simulink model "simulink_chapter_1"  (R2020b)
settings: Solver=VariableStepAuto  StartTime=0.0  StopTime=10.0  RelTol=1e-3
undefined symbols (not defined in the file): c, k, m
libraries: simulink x1
settings Model: Creator=yosef  LastModifiedBy=yosef

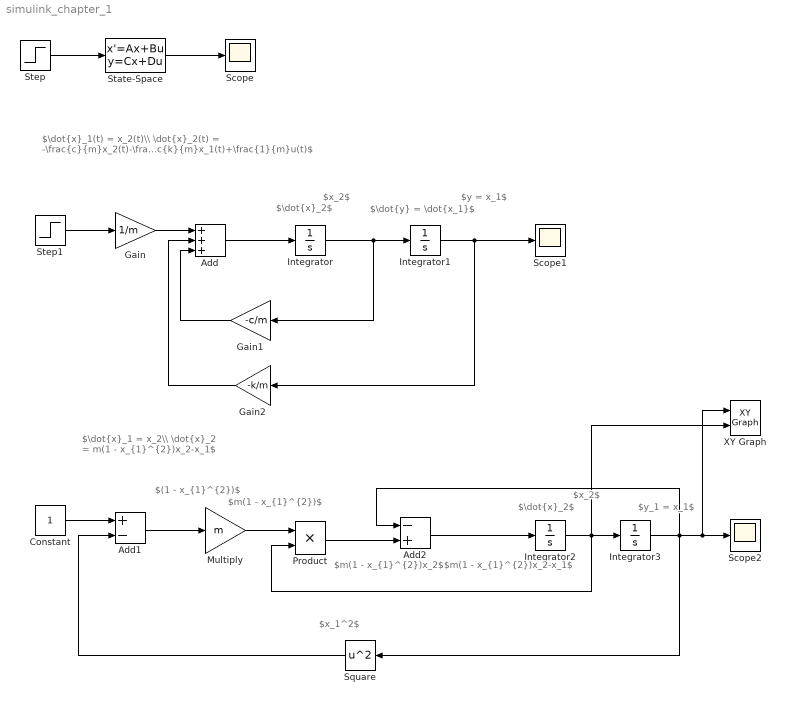
== system simulink_chapter_1 ==
  note: $\dot{x}_1(t) = x_2(t)\\ \dot{x}_2(t) = -\frac{c}{m}x_2(t)-\frac{k}{m}x_1(t)+\frac{1}{m}u(t)$
  note: $\dot{y} = \dot{x_1}$
  note: $y = x_1$
  note: $\dot{x}_2$
  note: $x_2$
  note: $\dot{x}_1 = x_2\\ \dot{x}_2 = m(1 - x_{1}^{2})x_2-x_1$
  note: $\dot{x}_2$
  note: $x_2$
  note: $y_1 = x_1$
  note: $x_1^2$
  note: $(1 - x_{1}^{2})$
  note: $m(1 - x_{1}^{2})$
  note: $m(1 - x_{1}^{2})x_2$
  note: $m(1 - x_{1}^{2})x_2-x_1$
  Add : Sum  Inputs=+++
  Add1 : Sum  Inputs=+-
  Add2 : Sum  Inputs=-+
  Constant : Constant
  Gain : Gain  Gain=1/m
  Gain1 : Gain  Gain=-c/m
  Gain2 : Gain  Gain=-k/m
  Integrator : Integrator
  Integrator1 : Integrator
  Integrator2 : Integrator  InitialCondition=2
  Integrator3 : Integrator  InitialCondition=1
  Multiply : Gain  Gain=m
  Product : Product
  Scope : Scope
  Scope1 : Scope
  Scope2 : Scope
  Square : Math  Operator=square  SaturateOnIntegerOverflow=on
  State-Space : StateSpace  A=[0 1; -0.5 -1.5]  B=[0; 0.5]  C=[1,0]  D=0  InitialCondition=0
  Step : Step  Time=0  SampleTime=0
  Step1 : Step  Time=0  SampleTime=0
  XY Graph : simulink/Sinks/XY Graph  xmin=-10  xmax=10  ymin=-3  ymax=3  st=-1
  wires:
  State-Space/1 -> Scope/1
  Step/1 -> State-Space/1
  Integrator/1 -> Gain1/1, Integrator1/1
  Add/1 -> Integrator/1
  Gain/1 -> Add/1
  Integrator1/1 -> Scope1/1, Gain2/1
  Gain1/1 -> Add/3
  Gain2/1 -> Add/2
  Step1/1 -> Gain/1
  Constant/1 -> Add1/1
  Integrator2/1 -> XY Graph/2, Product/2, Integrator3/1
  Product/1 -> Add2/2
  Add2/1 -> Integrator2/1
  Integrator3/1 -> Square/1, Add2/1, XY Graph/1, Scope2/1
  Multiply/1 -> Product/1
  Add1/1 -> Multiply/1
  Square/1 -> Add1/2
